simulink model "DCMotor"  (R2023a)
settings: Solver=VariableStepAuto  StartTime=0.0  StopTime=10.0  RelTol=1e-3
settings Model: Creator=dervint  LastModifiedBy=dervint

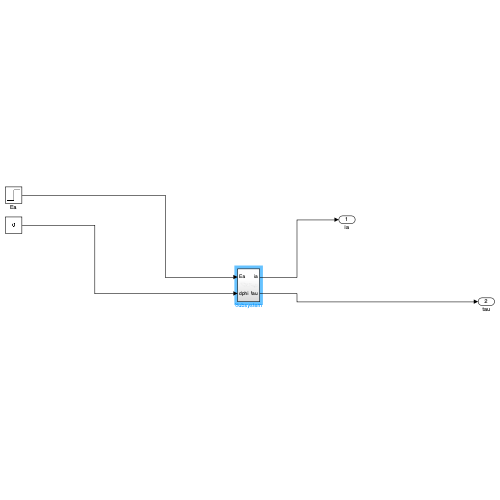
[thumbnail: Simulink's stored preview of the top-level diagram]
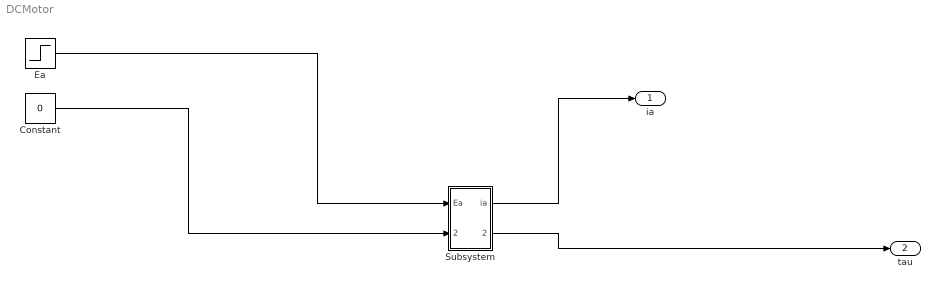
== system DCMotor ==
  Constant : Constant  Value=0
  Ea : Step  After=12  SampleTime=0
  Subsystem : Subsystem
  ia : Outport
  tau : Outport  Port=2
  wires:
  Ea/1 -> Subsystem/1(Ea)
  Constant/1 -> Subsystem/2(dphi)
  Subsystem/1(ia) -> ia/1
  Subsystem/2(tau) -> tau/1

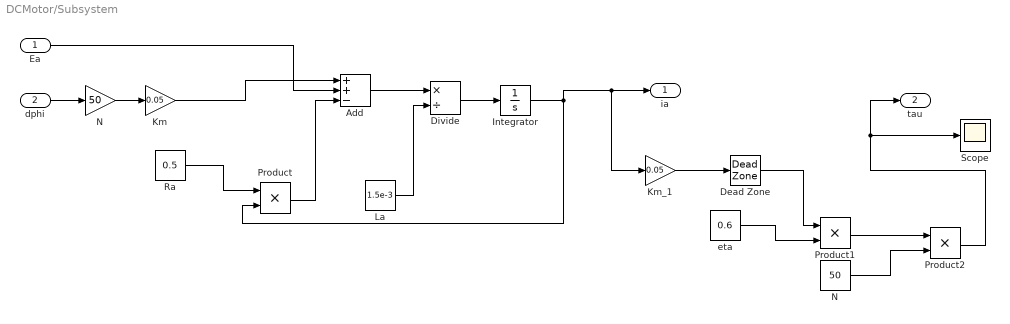
== system DCMotor/Subsystem ==
  Ea : Inport
  dphi : Inport  Port=2
  Add : Sum  Inputs=++-
  Dead Zone : DeadZone
  Divide : Product  Inputs=*/
  Integrator : Integrator
  Km : Gain  Gain=0.05
  Km_1 : Gain  Gain=0.05
  La : Constant  Value=1.5e-3
  N : Constant  Value=50
  "N " : Gain  Gain=50
  Product : Product
  Product1 : Product
  Product2 : Product
  Ra : Constant  Value=0.5
  Scope : Scope
  eta : Constant  Value=0.6
  ia : Outport
  tau : Outport  Port=2
  wires:
  Ea/1 -> Add/2
  Product1/1 -> Product2/1
  Km_1/1 -> Dead Zone/1
  dphi/1 -> "N "/1
  eta/1 -> Product1/2
  Add/1 -> Divide/1
  Dead Zone/1 -> Product1/1
  Integrator/1 -> ia/1, Km_1/1, Product/2
  "N "/1 -> Km/1
  Product/1 -> Add/3
  Km/1 -> Add/1
  N/1 -> Product2/2
  Ra/1 -> Product/1
  Product2/1 -> tau/1, Scope/1
  Divide/1 -> Integrator/1
  La/1 -> Divide/2
